simulink model "test"  (R2022b)
settings: Solver=ode23t  StartTime=0.0  StopTime=inf  FixedStep=1E-4  MaxStep=100  RelTol=1e-4  EnableMultiTasking=on
InitFcn:
  | iniASU_UNIT
model workspace (MAT data in the model file):
  Port = 10001
  Port2 = 50001
  RemoteIP = '0.0.0.0'
libraries: dspnetwork x7
settings Model: Creator=iirizar  LastModifiedBy=goigl
settings SolverCC: InitialStep=1E-22  MaxConsecutiveMinStep=auto  AlgebraicLoopSolver=TrustRegion  SolverResetMethod=Robust
settings DataIOCC: LimitDataPoints=on  MaxDataPoints=1  SaveFinalState=on  SaveFormat=Array  SignalLoggingSaveFormat=ModelDataLogs  SaveOutput=off  SaveState=on  SignalLogging=off  SaveTime=off  ReturnWorkspaceOutputs=off
settings OptimizationCC: ExpressionDepthLimit=2147483647  LifeSpan=inf
settings DebuggingCC: UnderspecifiedInitializationDetection=Classic  MergeDetectMultiDrivingBlocksExec=none  SolverPrmCheckMsg=warning  FcnCallInpInsideContextMsg=warning  UnconnectedInputMsg=warning  UnconnectedOutputMsg=warning  UnconnectedLineMsg=warning  StateNameClashWarn=warning  SFUnexpectedBacktrackingDiag=warning  SFNoUnconditionalDefaultTransitionDiag=warning  SFExecutionAtInitializationDiag=none  SFMachineParentedDataDiag=warning  ArithmeticOperatorsInVariantConditions=warning
settings HardwareCC: ProdBitPerPointer=32  ProdBitPerSizeT=32  ProdBitPerPtrDiffT=32  ProdLargestAtomicFloat=None  ProdIntDivRoundTo=Undefined  ProdEndianess=Unspecified  ProdWordSize=32  ProdHWDeviceType=32-bit Generic
settings ModelReferenceCC: EnableRefExpFcnMdlSchedulingChecks=on  PropagateSignalLabelsOutOfModel=off
settings SFSimCC: SimUseLocalCustomCode=off  CustomCodeUndefinedFunction=UseInterfaceOnly
settings RTWCC: RTWUseLocalCustomCode=off  DLArmComputeVersion=19.05
settings CodeAppCC: StateflowObjectComments=on
settings GRTTargetCC: TargetLangStandard=C89/C90 (ANSI)  CombineOutputUpdateFcns=off  GRTInterface=on
settings ConfigComp: CovMetricSettings=dw  CovSaveCumulativeToWorkspaceVar=on  CovSaveSingleToWorkspaceVar=on  CovExternalEMLEnable=off

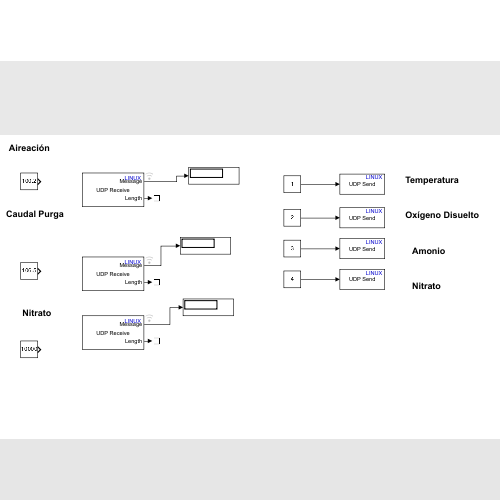
[thumbnail: Simulink's stored preview of the top-level diagram]
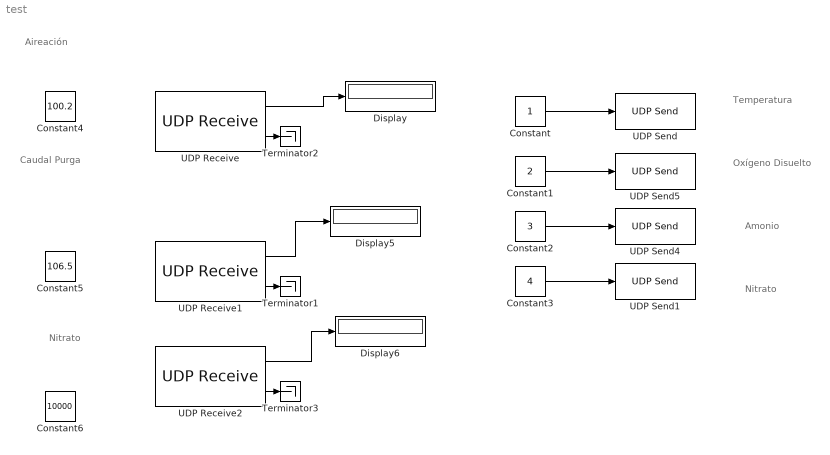
== system test ==
  note: Temperatura
  note: Oxígeno Disuelto
  note: Amonio
  note: Nitrato
  note: Aireación
  note: Caudal Purga
  note: Nitrato
  Constant : Constant
  Constant1 : Constant  Value=2
  Constant2 : Constant  Value=3
  Constant3 : Constant  Value=4
  Constant4 : Constant  Value=100.2
  Constant5 : Constant  Value=106.5
  Constant6 : Constant  Value=10000
  Display : Display
  Display5 : Display
  Display6 : Display
  Terminator1 : Terminator
  Terminator2 : Terminator
  Terminator3 : Terminator
  UDP Receive : dspnetwork/UDP Receive  localURL='0.0.0.0'  localPort=50001  remoteURL='localhost'  remotePort=-1  recvBufferSize=2  dims=1  signalDatatype=uint16  isComplex=off  isVarSize=off  showBlockingTime=on  blockingTime=0  sampletime=0.1  blockPlatform=LINUX
  UDP Receive1 : dspnetwork/UDP Receive  localURL='0.0.0.0'  localPort=50001  remoteURL='localhost'  remotePort=-1  recvBufferSize=2  dims=1  signalDatatype=uint16  isComplex=off  isVarSize=off  showBlockingTime=on  blockingTime=0  sampletime=0.1  blockPlatform=LINUX
  UDP Receive2 : dspnetwork/UDP Receive  localURL='0.0.0.0'  localPort=50001  remoteURL='localhost'  remotePort=-1  recvBufferSize=2  dims=1  signalDatatype=uint16  isComplex=off  isVarSize=off  showBlockingTime=on  blockingTime=0  sampletime=0.1  blockPlatform=LINUX
  UDP Send : dspnetwork/UDP Send  remoteURL='localhost'  remotePort=Port  localURL='255.255.255.255'  localPortSource=Automatically determine  localPort=-1  sendBufferSize=8192*2  sampletime=-1  blockPlatform=LINUX  separateLengthPort=0
  UDP Send1 : dspnetwork/UDP Send  remoteURL='localhost'  remotePort=Port+3  localURL='255.255.255.255'  localPortSource=Automatically determine  localPort=-1  sendBufferSize=8192*2  sampletime=-1  blockPlatform=LINUX  separateLengthPort=0
  UDP Send4 : dspnetwork/UDP Send  remoteURL='localhost'  remotePort=Port+2  localURL='255.255.255.255'  localPortSource=Automatically determine  localPort=-1  sendBufferSize=8192*2  sampletime=-1  blockPlatform=LINUX  separateLengthPort=0
  UDP Send5 : dspnetwork/UDP Send  remoteURL='localhost'  remotePort=Port+1  localURL='255.255.255.255'  localPortSource=Automatically determine  localPort=-1  sendBufferSize=8192*2  sampletime=-1  blockPlatform=LINUX  separateLengthPort=0
  wires:
  UDP Receive1/2 -> Terminator1/1
  UDP Receive2/2 -> Terminator3/1
  UDP Receive/2 -> Terminator2/1
  UDP Receive/1 -> Display/1
  UDP Receive1/1 -> Display5/1
  UDP Receive2/1 -> Display6/1
  Constant/1 -> UDP Send/1
  Constant1/1 -> UDP Send5/1
  Constant2/1 -> UDP Send4/1
  Constant3/1 -> UDP Send1/1
